simulink model "washingmachine"  (R2024b)
settings: Solver=VariableStepAuto  StartTime=0.0  StopTime=inf  RelTol=1e-3
settings Model: Creator=vivan  LastModifiedBy=vivan

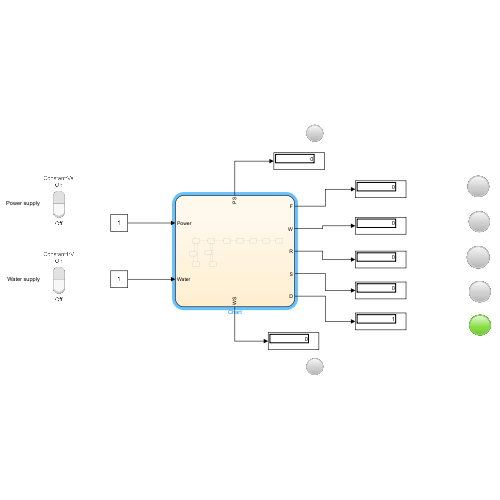
[thumbnail: Simulink's stored preview of the top-level diagram]
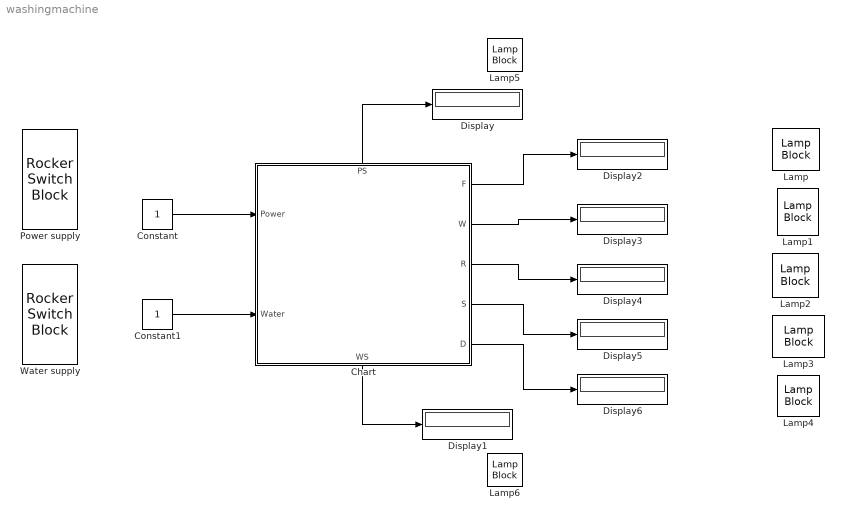
== system washingmachine ==
  Chart : Stateflow chart  TreatAsAtomicUnit=on
      settings: PortSchema="{\"entries\":[{\"content\":{\"sides\":[{\"content\":{\"connectorIds\":[\"In1\",\"In2\"]},\"type\":\"ConnectorPlacement.EquallySpacedRectSide\",\"uuid\":\"d7032c30-51a8-4fc2-9408-fe0addc3d492\"},{\"content\":{\"connectorIds\":[\"Out5\",\"Out6\",\"Out2\",\"Out1\",\"Out4\"],\"side\":\"RIGHT\"},\"type\":\"ConnectorPlacement.EquallySpacedRectSide\",\"uuid\":\"f7dc864a-3893-4283-9c39-66f45ca5cd1b\"},{\"content\":{\"connectorIds\":[\"Out3\"],\"side\":\"TOP\"},\"type\":\"ConnectorPlacement.EquallySpacedRectSide\",\"uuid\":\"ebf97e33-4f03-43bf-aa31-1cc0b2db0caa\"},{\"content\":{\"connectorIds\":[\"Out7\"],\"side\":\"BOTTOM\"},\"type\":\"ConnectorPlacement.EquallySpacedRectSide\",\"uuid\":\"f12e8b74-efbd-4917-900c-eaf7d683c120\"}]},\"type\":\"ConnectorPlacement.EquallySpacedConnector\",\"uuid\":\"8b45bfa7-581d-4e60-9a5f-6c29c44be655\"}],\"packageUris\":[\"http://schema.mathworks.com/mf0/Connector/R2020b\"],\"version\":\"1.0\"}"
  Constant : Constant
  Constant1 : Constant
  Display{,1..6} (7 alike) : Display
  Lamp{,1..6} (7 alike) : LampBlock  LabelPosition=Hide
  Power supply : RockerSwitchBlock
      settings: Values={{'Off', 'On'}, [0 1]}
  Water supply : RockerSwitchBlock
      settings: Values={{'Off', 'On'}, [0 1]}
  wires:
  Constant/1 -> Chart/1(Power)
  Constant1/1 -> Chart/2(Water)
  Chart/3(PS) -> Display/1
  Chart/5(F) -> Display2/1
  Chart/6(W) -> Display3/1
  Chart/2(R) -> Display4/1
  Chart/1(S) -> Display5/1
  Chart/4(D) -> Display6/1
  Chart/7(WS) -> Display1/1

== stateflow chart washingmachine/Chart ==
  state Filling
    entry:F=1;
  state Washing
    entry:F=0,W=1;
  state Rinsing
    entry:W=0,R=1;
  state Power_Supply
  state Water_Supply
  state Spining
    entry:R=0,S=1;
  state Done
    entry:S=0,D=1;
  state Water_Indicator1
    entry:WS=0
  state Power_indicator1
    entry:PS=0
  state Power_indicator
    entry:PS=1
  state Water_Indicator
    entry:WS=1
  (default) -> Power_Supply
  Water_Supply -> Filling [order 1] : [Water==1]
  Filling -> Washing : [after(10,sec)]
  Washing -> Rinsing : [after(10,sec)]
  Rinsing -> Spining : [after(10,sec)]
  Power_Supply -> Water_Supply [order 1] : [Power==1]
  Spining -> Done : [after(10,sec)]
  Power_indicator1 -> Power_Supply : [Power==1]
  Power_Supply -> Power_indicator [order 2] : [Power==0]
  Water_Indicator1 -> Water_Supply : [Water==1]
  Water_Supply -> Water_Indicator [order 2] : [Water==0]
  Water_Indicator -> Water_Indicator1 : [Water==1]
  Power_indicator -> Power_indicator1 : [Power==1]
  data: Power input; Water input; S output; R output; PS output; D output; F output; W output; WS output
